simulink model "Aufgabe11_Vorlage_Prozessgut"  (R2022a)
settings: Solver=ode3  StartTime=0.0  StopTime=50  RelTol=1e-3  EnableMultiTasking=on
undefined symbols (not defined in the file): MaxFlaschen
libraries: simulink x19
settings Model: Creator=merz  LastModifiedBy=60251
settings SolverCC: ZeroCrossAlgorithm=Non-adaptive  AlgebraicLoopSolver=TrustRegion
settings DataIOCC: LimitDataPoints=on  SaveFormat=Array  SignalLoggingSaveFormat=ModelDataLogs  ReturnWorkspaceOutputs=off  SignalLoggingName=sigsOut
settings OptimizationCC: ExpressionDepthLimit=2147483647  InitFltsAndDblsToZero=on  LifeSpan=inf
settings DebuggingCC: SaveWithParameterizedLinksMsg=none  UnderspecifiedInitializationDetection=Classic  MergeDetectMultiDrivingBlocksExec=none  SignalResolutionControl=TryResolveAllWithWarning  MultiTaskDSMMsg=warning  MultiTaskCondExecSysMsg=none  FcnCallInpInsideContextMsg=warning  UnconnectedInputMsg=warning  UnconnectedOutputMsg=warning  UnconnectedLineMsg=warning  StateNameClashWarn=warning  SFUnexpectedBacktrackingDiag=warning  SFNoUnconditionalDefaultTransitionDiag=warning  SFExecutionAtInitializationDiag=none  SFMachineParentedDataDiag=warning  ArithmeticOperatorsInVariantConditions=warning
settings HardwareCC: ProdBitPerPointer=32  ProdBitPerSizeT=32  ProdBitPerPtrDiffT=32  ProdLargestAtomicFloat=None  ProdIntDivRoundTo=Undefined  ProdEndianess=Unspecified  ProdWordSize=32  ProdHWDeviceType=32-bit Generic  TargetUnknown=on
settings ModelReferenceCC: PropagateSignalLabelsOutOfModel=off
settings RTWCC: DLArmComputeVersion=19.05
settings CodeAppCC: StateflowObjectComments=on
settings GRTTargetCC: TargetFcnLib=ansi_tfl_tmw.mat  TargetLangStandard=C89/C90 (ANSI)  ModelReferenceCompliant=off  CombineOutputUpdateFcns=off  MatFileLogging=off  GRTInterface=on
settings ConfigComp: CovMetricSettings=dw  CovSaveCumulativeToWorkspaceVar=on  CovSaveSingleToWorkspaceVar=on

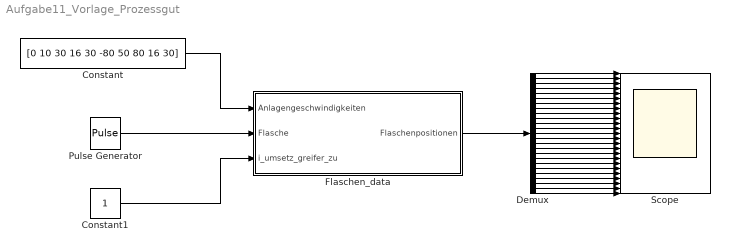
== system Aufgabe11_Vorlage_Prozessgut ==
  Constant : Constant  Value=[0 10 30 16 30 -80 50 80 16 30]
  Constant1 : Constant
  Demux : Demux  Outputs=25
  Flaschen_data : Subsystem
  Pulse Generator : DiscretePulseGenerator  PulseType=Time based  Period=3  PulseWidth=10
  Scope : Scope  NumInputPorts=25
  wires:
  Constant/1 -> Flaschen_data/1(Anlagengeschwindigkeiten)
  Constant1/1 -> Flaschen_data/3(i_umsetz_greifer_zu)
  Flaschen_data/1(Flaschenpositionen) -> Demux/1
  Demux/1 -> Scope/1
  Demux/2 -> Scope/2
  Demux/3 -> Scope/3
  Demux/4 -> Scope/4
  Demux/5 -> Scope/5
  Demux/6 -> Scope/6
  Demux/7 -> Scope/7
  Demux/8 -> Scope/8
  Demux/9 -> Scope/9
  Demux/10 -> Scope/10
  Demux/11 -> Scope/11
  Demux/12 -> Scope/12
  Demux/13 -> Scope/13
  Demux/14 -> Scope/14
  Demux/15 -> Scope/15
  Demux/16 -> Scope/16
  Demux/17 -> Scope/17
  Demux/18 -> Scope/18
  Demux/19 -> Scope/19
  Demux/20 -> Scope/20
  Demux/21 -> Scope/21
  Demux/22 -> Scope/22
  Demux/23 -> Scope/23
  Demux/24 -> Scope/24
  Demux/25 -> Scope/25
  Pulse Generator/1 -> Flaschen_data/2(Flasche)

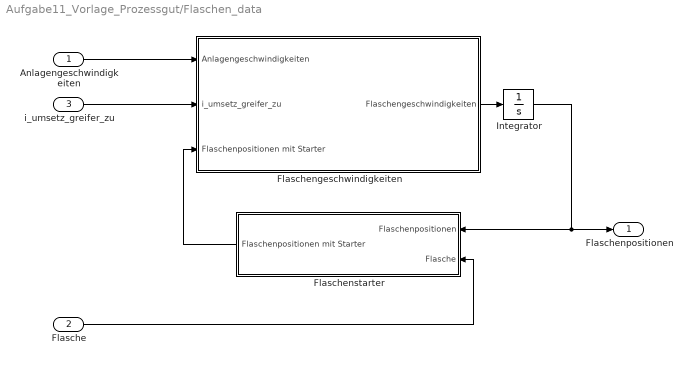
== system Aufgabe11_Vorlage_Prozessgut/Flaschen_data ==
  Anlagengeschwindigkeiten : Inport
  Flasche : Inport  Port=2
  i_umsetz_greifer_zu : Inport  Port=3
  Flaschengeschwindigkeiten : Subsystem
  Flaschenstarter : Subsystem
  Integrator : Integrator
  Flaschenpositionen : Outport
  wires:
  Flasche/1 -> Flaschenstarter/2(Flasche)
  Flaschenstarter/1(Flaschenpositionen mit Starter) -> Flaschengeschwindigkeiten/3(Flaschenpositionen mit Starter)
  i_umsetz_greifer_zu/1 -> Flaschengeschwindigkeiten/2(i_umsetz_greifer_zu)
  Anlagengeschwindigkeiten/1 -> Flaschengeschwindigkeiten/1(Anlagengeschwindigkeiten)
  Flaschengeschwindigkeiten/1(Flaschengeschwindigkeiten) -> Integrator/1
  Integrator/1 -> Flaschenstarter/1(Flaschenpositionen), Flaschenpositionen/1

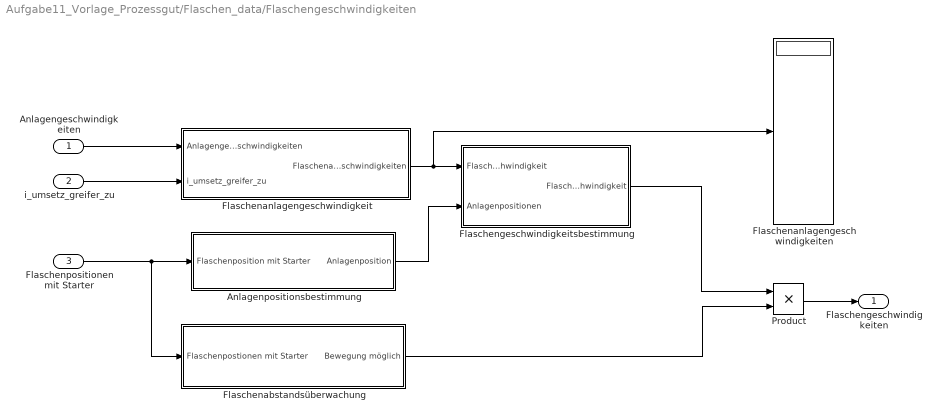
== system Aufgabe11_Vorlage_Prozessgut/Flaschen_data/Flaschengeschwindigkeiten ==
  Anlagengeschwindigkeiten : Inport
  i_umsetz_greifer_zu : Inport  Port=2
  Flaschenpositionen mit Starter : Inport  Port=3
  Anlagenpositionsbestimmung : Subsystem
  Flaschenabstandsüberwachung : Subsystem
  Flaschenanlagengeschwindigkeit : Subsystem
  Flaschenanlagengeschwindigkeiten : Display
  "Flaschengeschwindigkeitsbestimmung " : Subsystem  TreatAsAtomicUnit=on
  Product : Product
  Flaschengeschwindigkeiten : Outport
  wires:
  Anlagengeschwindigkeiten/1 -> Flaschenanlagengeschwindigkeit/1(Anlagengeschwindigkeiten)
  i_umsetz_greifer_zu/1 -> Flaschenanlagengeschwindigkeit/2(i_umsetz_greifer_zu)
  Flaschenpositionen mit Starter/1 -> Flaschenabstandsüberwachung/1(Flaschenpostionen mit Starter), Anlagenpositionsbestimmung/1(Flaschenposition mit Starter)
  Flaschenanlagengeschwindigkeit/1(Flaschenanlagengeschwindigkeiten) -> Flaschenanlagengeschwindigkeiten/1, "Flaschengeschwindigkeitsbestimmung "/1(Flaschenanlagengeschwindigkeit)
  Product/1 -> Flaschengeschwindigkeiten/1
  Flaschenabstandsüberwachung/1(Bewegung möglich) -> Product/2
  "Flaschengeschwindigkeitsbestimmung "/1(Flaschengeschwindigkeit) -> Product/1
  Anlagenpositionsbestimmung/1(Anlagenposition) -> "Flaschengeschwindigkeitsbestimmung "/2(Anlagenpositionen)

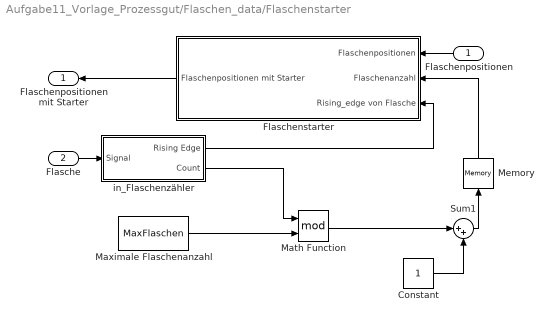
== system Aufgabe11_Vorlage_Prozessgut/Flaschen_data/Flaschenstarter ==
  Flaschenpositionen : Inport
  Flasche : Inport  Port=2
  Constant : Constant  OutDataTypeStr=uint16
  Flaschenstarter : Subsystem
  Math Function : Math  Operator=mod  SignedPower=on
  Maximale Flaschenanzahl : Constant  Value=MaxFlaschen  OutDataTypeStr=uint16
  Memory : Memory  InitialCondition=1
  Sum1 : Sum  Inputs=|++  SaturateOnIntegerOverflow=on
  in_Flaschenzähler : Subsystem
  Flaschenpositionen mit Starter : Outport
  wires:
  in_Flaschenzähler/2(Count) -> Math Function/1
  Maximale Flaschenanzahl/1 -> Math Function/2
  Math Function/1 -> Sum1/1
  in_Flaschenzähler/1(Rising Edge) -> Flaschenstarter/3(Rising_edge von Flasche)
  Sum1/1 -> Memory/1
  Constant/1 -> Sum1/2
  Memory/1 -> Flaschenstarter/2(Flaschenanzahl)
  Flaschenpositionen/1 -> Flaschenstarter/1(Flaschenpositionen)
  Flaschenstarter/1(Flaschenpositionen mit Starter) -> Flaschenpositionen mit Starter/1
  Flasche/1 -> in_Flaschenzähler/1(Signal)

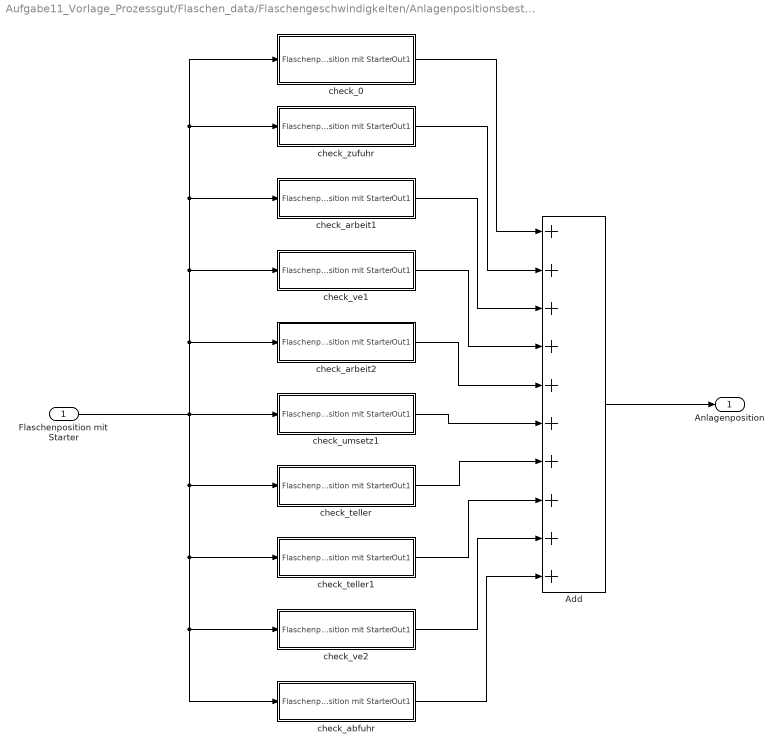
== system Aufgabe11_Vorlage_Prozessgut/Flaschen_data/Flaschengeschwindigkeiten/Anlagenpositionsbestimmung ==
  Flaschenposition mit Starter : Inport
  Add : Sum  Inputs=++++++++++
  check_0 : Subsystem
  check_abfuhr : Subsystem
  check_arbeit1 : Subsystem
  check_arbeit2 : Subsystem
  check_teller : Subsystem
  check_teller1 : Subsystem
  check_umsetz1 : Subsystem
  check_ve1 : Subsystem
  check_ve2 : Subsystem
  check_zufuhr : Subsystem
  Anlagenposition : Outport
  wires:
  Add/1 -> Anlagenposition/1
  Flaschenposition mit Starter/1 -> check_abfuhr/1(Flaschenposition mit Starter), check_ve2/1(Flaschenposition mit Starter), check_teller1/1(Flaschenposition mit Starter), check_teller/1(Flaschenposition mit Starter), check_0/1(Flaschenposition mit Starter), check_zufuhr/1(Flaschenposition mit Starter), check_arbeit1/1(Flaschenposition mit Starter), check_ve1/1(Flaschenposition mit Starter), check_arbeit2/1(Flaschenposition mit Starter), check_umsetz1/1(Flaschenposition mit Starter)
  check_umsetz1/1(Out1) -> Add/6
  check_teller/1(Out1) -> Add/7
  check_arbeit2/1(Out1) -> Add/5
  check_teller1/1(Out1) -> Add/8
  check_ve1/1(Out1) -> Add/4
  check_ve2/1(Out1) -> Add/9
  check_arbeit1/1(Out1) -> Add/3
  check_abfuhr/1(Out1) -> Add/10
  check_zufuhr/1(Out1) -> Add/2
  check_0/1(Out1) -> Add/1

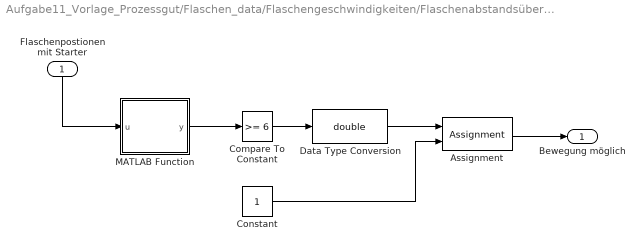
== system Aufgabe11_Vorlage_Prozessgut/Flaschen_data/Flaschengeschwindigkeiten/Flaschenabstandsüberwachung ==
  Flaschenpostionen mit Starter : Inport
  Assignment : Assignment  DiagnosticForDimensions=Warning  IndexOptions=Index vector (dialog)  Indices=1  OutputSizes=1
  Compare To Constant : simulink/Logic and Bit Operations/Compare To Constant  relop=>=  const=6  OutDataTypeStr=boolean
  Constant : Constant
  Data Type Conversion : DataTypeConversion  OutDataTypeStr=double  SaturateOnIntegerOverflow=off  RndMeth=Floor
  MATLAB Function : MATLAB Function  TreatAsAtomicUnit=on
  Bewegung möglich : Outport
  wires:
  Flaschenpostionen mit Starter/1 -> MATLAB Function/1(u)
  MATLAB Function/1(y) -> Compare To Constant/1
  Compare To Constant/1 -> Data Type Conversion/1
  Data Type Conversion/1 -> Assignment/1
  Constant/1 -> Assignment/2
  Assignment/1 -> Bewegung möglich/1

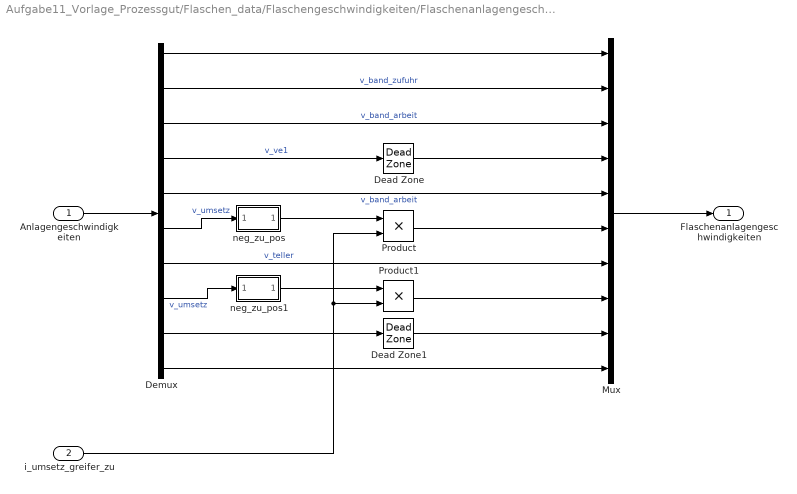
== system Aufgabe11_Vorlage_Prozessgut/Flaschen_data/Flaschengeschwindigkeiten/Flaschenanlagengeschwindigkeit ==
  Anlagengeschwindigkeiten : Inport
  i_umsetz_greifer_zu : Inport  Port=2
  Dead Zone : DeadZone  LowerValue=-inf  UpperValue=0
  Dead Zone1 : DeadZone  LowerValue=-inf  UpperValue=0
  Demux : Demux  Outputs=10
  Mux : Mux  Inputs=10
  Product : Product
  Product1 : Product
  neg_zu_pos : Subsystem
  neg_zu_pos1 : Subsystem
  Flaschenanlagengeschwindigkeiten : Outport
  wires:
  Anlagengeschwindigkeiten/1 -> Demux/1
  Mux/1 -> Flaschenanlagengeschwindigkeiten/1
  Demux/1 -> Mux/1
  Demux/2 -> Mux/2  "v_band_zufuhr"
  Demux/3 -> Mux/3  "v_band_arbeit"
  Demux/4 -> Dead Zone/1  "v_ve1"
  Dead Zone/1 -> Mux/4
  Demux/5 -> Mux/5  "v_band_arbeit"
  Product/1 -> Mux/6
  Demux/6 -> neg_zu_pos/1(In1)  "v_umsetz"
  neg_zu_pos/1(Out1) -> Product/1
  i_umsetz_greifer_zu/1 -> Product/2, Product1/2
  neg_zu_pos1/1(Out1) -> Product1/1
  Demux/7 -> Mux/7  "v_teller"
  Demux/8 -> neg_zu_pos1/1(In1)  "v_umsetz"
  Demux/10 -> Mux/10
  Demux/9 -> Dead Zone1/1
  Product1/1 -> Mux/8
  Dead Zone1/1 -> Mux/9

== system Aufgabe11_Vorlage_Prozessgut/Flaschen_data/Flaschengeschwindigkeiten/Flaschengeschwindigkeitsbestimmung  ==
  Flaschenanlagengeschwindigkeit : Inport
  Anlagenpositionen : Inport  Port=2
  Selector : Selector  InputPortWidth=10  IndexOptions=Index vector (port)  Indices=[1 3]  OutputSizes=1
  Flaschengeschwindigkeit : Outport
  wires:
  Anlagenpositionen/1 -> Selector/2
  Flaschenanlagengeschwindigkeit/1 -> Selector/1
  Selector/1 -> Flaschengeschwindigkeit/1

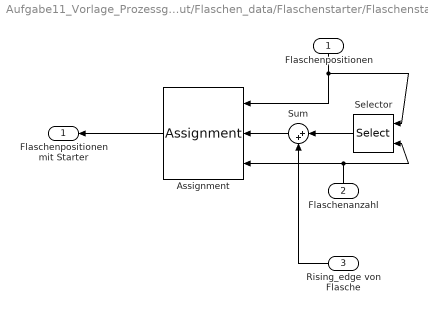
== system Aufgabe11_Vorlage_Prozessgut/Flaschen_data/Flaschenstarter/Flaschenstarter ==
  Flaschenpositionen : Inport
  Flaschenanzahl : Inport  Port=2
  Rising_edge von Flasche : Inport  Port=3
  Assignment : Assignment  IndexOptions=Index vector (port)  Indices=1  OutputSizes=[1]
  Selector : Selector  InputPortWidth=MaxFlaschen  IndexOptions=Index vector (port)  Indices=[1 3]  OutputSizes=1
  Sum : Sum  Inputs=|++  OutDataTypeStr=double  RndMeth=Zero
  Flaschenpositionen mit Starter : Outport
  wires:
  Selector/1 -> Sum/1
  Sum/1 -> Assignment/2
  Flaschenanzahl/1 -> Selector/2, Assignment/3
  Flaschenpositionen/1 -> Assignment/1, Selector/1
  Assignment/1 -> Flaschenpositionen mit Starter/1
  Rising_edge von Flasche/1 -> Sum/2

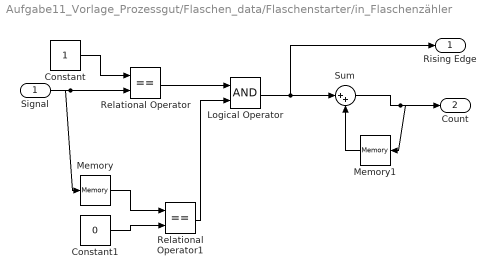
== system Aufgabe11_Vorlage_Prozessgut/Flaschen_data/Flaschenstarter/in_Flaschenzähler ==
  Signal : Inport
  Constant : Constant
  Constant1 : Constant  Value=0
  Logical Operator : Logic  AllPortsSameDT=off
  Memory : Memory
  Memory1 : Memory
  Relational Operator : RelationalOperator  Operator===  InputSameDT=off
  Relational Operator1 : RelationalOperator  Operator===  InputSameDT=off
  Sum : Sum  Inputs=|++  OutDataTypeStr=uint16  SaturateOnIntegerOverflow=on
  Rising Edge : Outport
  Count : Outport  Port=2
  wires:
  Signal/1 -> Memory/1, Relational Operator/2
  Constant/1 -> Relational Operator/1
  Relational Operator/1 -> Logical Operator/1
  Constant1/1 -> Relational Operator1/2
  Memory/1 -> Relational Operator1/1
  Relational Operator1/1 -> Logical Operator/2
  Logical Operator/1 -> Sum/1, Rising Edge/1
  Memory1/1 -> Sum/2
  Sum/1 -> Count/1, Memory1/1

== system Aufgabe11_Vorlage_Prozessgut/Flaschen_data/Flaschengeschwindigkeiten/Anlagenpositionsbestimmung/check_0 ==
  Flaschenposition mit Starter : Inport
  Compare To Constant : simulink/Logic and Bit Operations/Compare To Constant  relop===  const=0  OutDataTypeStr=boolean
  Data Type Conversion : DataTypeConversion  OutDataTypeStr=double  SaturateOnIntegerOverflow=off  RndMeth=Floor
  Out1 : Outport
  wires:
  Flaschenposition mit Starter/1 -> Compare To Constant/1
  Compare To Constant/1 -> Data Type Conversion/1
  Data Type Conversion/1 -> Out1/1

== system Aufgabe11_Vorlage_Prozessgut/Flaschen_data/Flaschengeschwindigkeiten/Anlagenpositionsbestimmung/check_abfuhr ==
  Flaschenposition mit Starter : Inport
  Compare To Constant1 : simulink/Logic and Bit Operations/Compare To Constant  relop=>=  const=610  OutDataTypeStr=boolean
  Data Type Conversion : DataTypeConversion  OutDataTypeStr=double  SaturateOnIntegerOverflow=off  RndMeth=Floor
  Gain : Gain  Gain=10
  Out1 : Outport
  wires:
  Gain/1 -> Out1/1
  Compare To Constant1/1 -> Data Type Conversion/1
  Flaschenposition mit Starter/1 -> Compare To Constant1/1
  Data Type Conversion/1 -> Gain/1

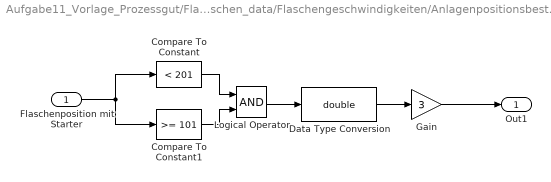
== system Aufgabe11_Vorlage_Prozessgut/Flaschen_data/Flaschengeschwindigkeiten/Anlagenpositionsbestimmung/check_arbeit1 ==
  Flaschenposition mit Starter : Inport
  Compare To Constant : simulink/Logic and Bit Operations/Compare To Constant  relop=<  const=201  OutDataTypeStr=boolean
  Compare To Constant1 : simulink/Logic and Bit Operations/Compare To Constant  relop=>=  const=101  OutDataTypeStr=boolean
  Data Type Conversion : DataTypeConversion  OutDataTypeStr=double  SaturateOnIntegerOverflow=off  RndMeth=Floor
  Gain : Gain  Gain=3
  Logical Operator : Logic  AllPortsSameDT=off  OutDataTypeStr=boolean
  Out1 : Outport
  wires:
  Data Type Conversion/1 -> Gain/1
  Flaschenposition mit Starter/1 -> Compare To Constant/1, Compare To Constant1/1
  Logical Operator/1 -> Data Type Conversion/1
  Compare To Constant1/1 -> Logical Operator/2
  Compare To Constant/1 -> Logical Operator/1
  Gain/1 -> Out1/1

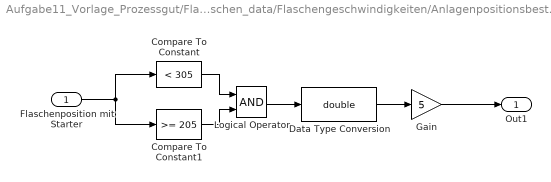
== system Aufgabe11_Vorlage_Prozessgut/Flaschen_data/Flaschengeschwindigkeiten/Anlagenpositionsbestimmung/check_arbeit2 ==
  Flaschenposition mit Starter : Inport
  Compare To Constant : simulink/Logic and Bit Operations/Compare To Constant  relop=<  const=305  OutDataTypeStr=boolean
  Compare To Constant1 : simulink/Logic and Bit Operations/Compare To Constant  relop=>=  const=205  OutDataTypeStr=boolean
  Data Type Conversion : DataTypeConversion  OutDataTypeStr=double  SaturateOnIntegerOverflow=off  RndMeth=Floor
  Gain : Gain  Gain=5
  Logical Operator : Logic  AllPortsSameDT=off  OutDataTypeStr=boolean
  Out1 : Outport
  wires:
  Data Type Conversion/1 -> Gain/1
  Flaschenposition mit Starter/1 -> Compare To Constant/1, Compare To Constant1/1
  Logical Operator/1 -> Data Type Conversion/1
  Compare To Constant1/1 -> Logical Operator/2
  Compare To Constant/1 -> Logical Operator/1
  Gain/1 -> Out1/1

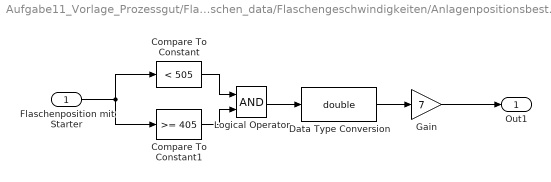
== system Aufgabe11_Vorlage_Prozessgut/Flaschen_data/Flaschengeschwindigkeiten/Anlagenpositionsbestimmung/check_teller ==
  Flaschenposition mit Starter : Inport
  Compare To Constant : simulink/Logic and Bit Operations/Compare To Constant  relop=<  const=505  OutDataTypeStr=boolean
  Compare To Constant1 : simulink/Logic and Bit Operations/Compare To Constant  relop=>=  const=405  OutDataTypeStr=boolean
  Data Type Conversion : DataTypeConversion  OutDataTypeStr=double  SaturateOnIntegerOverflow=off  RndMeth=Floor
  Gain : Gain  Gain=7
  Logical Operator : Logic  AllPortsSameDT=off  OutDataTypeStr=boolean
  Out1 : Outport
  wires:
  Data Type Conversion/1 -> Gain/1
  Flaschenposition mit Starter/1 -> Compare To Constant/1, Compare To Constant1/1
  Logical Operator/1 -> Data Type Conversion/1
  Compare To Constant1/1 -> Logical Operator/2
  Compare To Constant/1 -> Logical Operator/1
  Gain/1 -> Out1/1

== system Aufgabe11_Vorlage_Prozessgut/Flaschen_data/Flaschengeschwindigkeiten/Anlagenpositionsbestimmung/check_teller1 ==
  Flaschenposition mit Starter : Inport
  Compare To Constant : simulink/Logic and Bit Operations/Compare To Constant  relop=<  const=605  OutDataTypeStr=boolean
  Compare To Constant1 : simulink/Logic and Bit Operations/Compare To Constant  relop=>=  const=505  OutDataTypeStr=boolean
  Data Type Conversion : DataTypeConversion  OutDataTypeStr=double  SaturateOnIntegerOverflow=off  RndMeth=Floor
  Gain : Gain  Gain=8
  Logical Operator : Logic  AllPortsSameDT=off  OutDataTypeStr=boolean
  Out1 : Outport
  wires:
  Gain/1 -> Out1/1
  Compare To Constant/1 -> Logical Operator/1
  Compare To Constant1/1 -> Logical Operator/2
  Logical Operator/1 -> Data Type Conversion/1
  Flaschenposition mit Starter/1 -> Compare To Constant1/1, Compare To Constant/1
  Data Type Conversion/1 -> Gain/1

== system Aufgabe11_Vorlage_Prozessgut/Flaschen_data/Flaschengeschwindigkeiten/Anlagenpositionsbestimmung/check_umsetz1 ==
  Flaschenposition mit Starter : Inport
  Compare To Constant : simulink/Logic and Bit Operations/Compare To Constant  relop=<  const=405  OutDataTypeStr=boolean
  Compare To Constant1 : simulink/Logic and Bit Operations/Compare To Constant  relop=>=  const=305  OutDataTypeStr=boolean
  Data Type Conversion : DataTypeConversion  OutDataTypeStr=double  SaturateOnIntegerOverflow=off  RndMeth=Floor
  Gain : Gain  Gain=6
  Logical Operator : Logic  AllPortsSameDT=off  OutDataTypeStr=boolean
  Out1 : Outport
  wires:
  Gain/1 -> Out1/1
  Compare To Constant/1 -> Logical Operator/1
  Compare To Constant1/1 -> Logical Operator/2
  Logical Operator/1 -> Data Type Conversion/1
  Flaschenposition mit Starter/1 -> Compare To Constant1/1, Compare To Constant/1
  Data Type Conversion/1 -> Gain/1

== system Aufgabe11_Vorlage_Prozessgut/Flaschen_data/Flaschengeschwindigkeiten/Anlagenpositionsbestimmung/check_ve1 ==
  Flaschenposition mit Starter : Inport
  Compare To Constant : simulink/Logic and Bit Operations/Compare To Constant  relop=<  const=205  OutDataTypeStr=boolean
  Compare To Constant1 : simulink/Logic and Bit Operations/Compare To Constant  relop=>=  const=201  OutDataTypeStr=boolean
  Data Type Conversion : DataTypeConversion  OutDataTypeStr=double  SaturateOnIntegerOverflow=off  RndMeth=Floor
  Gain : Gain  Gain=4
  Logical Operator : Logic  AllPortsSameDT=off  OutDataTypeStr=boolean
  Out1 : Outport
  wires:
  Gain/1 -> Out1/1
  Compare To Constant/1 -> Logical Operator/1
  Compare To Constant1/1 -> Logical Operator/2
  Logical Operator/1 -> Data Type Conversion/1
  Flaschenposition mit Starter/1 -> Compare To Constant1/1, Compare To Constant/1
  Data Type Conversion/1 -> Gain/1

== system Aufgabe11_Vorlage_Prozessgut/Flaschen_data/Flaschengeschwindigkeiten/Anlagenpositionsbestimmung/check_ve2 ==
  Flaschenposition mit Starter : Inport
  Compare To Constant : simulink/Logic and Bit Operations/Compare To Constant  relop=<  const=610  OutDataTypeStr=boolean
  Compare To Constant1 : simulink/Logic and Bit Operations/Compare To Constant  relop=>=  const=605  OutDataTypeStr=boolean
  Data Type Conversion : DataTypeConversion  OutDataTypeStr=double  SaturateOnIntegerOverflow=off  RndMeth=Floor
  Gain : Gain  Gain=9
  Logical Operator : Logic  AllPortsSameDT=off  OutDataTypeStr=boolean
  Out1 : Outport
  wires:
  Data Type Conversion/1 -> Gain/1
  Flaschenposition mit Starter/1 -> Compare To Constant/1, Compare To Constant1/1
  Logical Operator/1 -> Data Type Conversion/1
  Compare To Constant1/1 -> Logical Operator/2
  Compare To Constant/1 -> Logical Operator/1
  Gain/1 -> Out1/1

== system Aufgabe11_Vorlage_Prozessgut/Flaschen_data/Flaschengeschwindigkeiten/Anlagenpositionsbestimmung/check_zufuhr ==
  Flaschenposition mit Starter : Inport
  Compare To Constant : simulink/Logic and Bit Operations/Compare To Constant  relop=<  const=101  OutDataTypeStr=boolean
  Compare To Constant1 : simulink/Logic and Bit Operations/Compare To Constant  relop=>  const=0  OutDataTypeStr=boolean
  Data Type Conversion : DataTypeConversion  OutDataTypeStr=double  SaturateOnIntegerOverflow=off  RndMeth=Floor
  Gain : Gain  Gain=2
  Logical Operator : Logic  AllPortsSameDT=off  OutDataTypeStr=boolean
  Out1 : Outport
  wires:
  Compare To Constant/1 -> Logical Operator/1
  Compare To Constant1/1 -> Logical Operator/2
  Logical Operator/1 -> Data Type Conversion/1
  Flaschenposition mit Starter/1 -> Compare To Constant1/1, Compare To Constant/1
  Data Type Conversion/1 -> Gain/1
  Gain/1 -> Out1/1

== system Aufgabe11_Vorlage_Prozessgut/Flaschen_data/Flaschengeschwindigkeiten/Flaschenanlagengeschwindigkeit/neg_zu_pos ==
  In1 : Inport
  Abs : Abs  SaturateOnIntegerOverflow=off
  Add : Sum  Inputs=-+
  Gain : Gain  Gain=.5
  Out1 : Outport
  wires:
  In1/1 -> Add/1, Abs/1
  Abs/1 -> Add/2
  Gain/1 -> Out1/1
  Add/1 -> Gain/1

== system Aufgabe11_Vorlage_Prozessgut/Flaschen_data/Flaschengeschwindigkeiten/Flaschenanlagengeschwindigkeit/neg_zu_pos1 ==
  In1 : Inport
  Abs : Abs  SaturateOnIntegerOverflow=off
  Add : Sum
  Gain : Gain  Gain=.5
  Out1 : Outport
  wires:
  Add/1 -> Gain/1
  Gain/1 -> Out1/1
  Abs/1 -> Add/2
  In1/1 -> Abs/1, Add/1

== matlab function Aufgabe11_Vorlage_Prozessgut/Flaschen_data/Flaschengeschwindigkeiten/Flaschenabstandsüberwachung/MATLAB Function ==
  data: u input; y output
function y = fcn(u)

y = circshift(u,1)-u;
